simulink model "Simulink_Driver_motor_BLDC"  (R2016a)
settings: Solver=VariableStepAuto  StartTime=0.0  StopTime=0.5  RelTol=1e-3
libraries: powerlib x12, powerlib_meascontrol x1
settings Model: Creator=COMPAQ  LastModifiedBy=COMPAQ

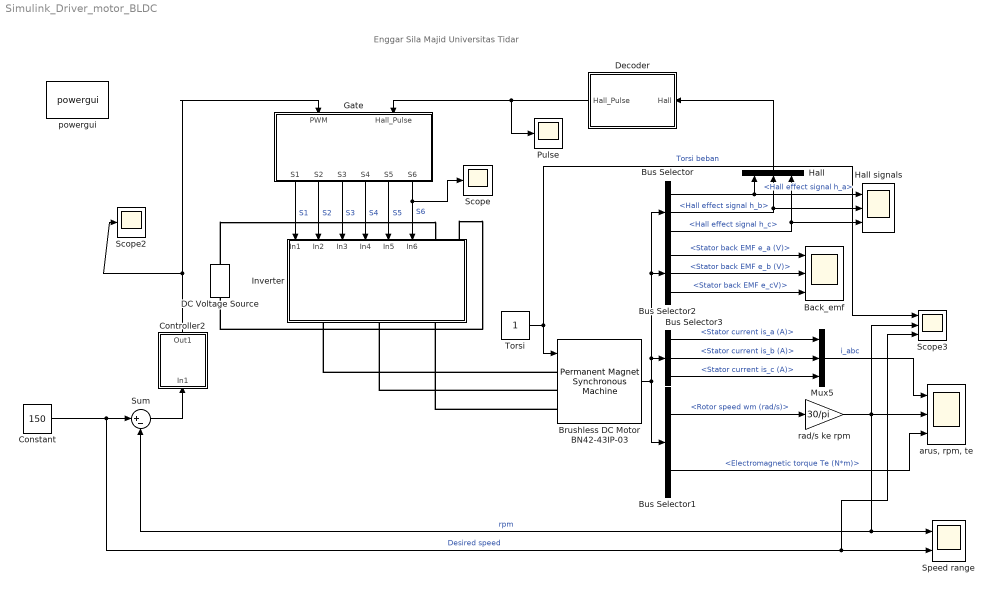
== system Simulink_Driver_motor_BLDC ==
  note: Enggar Sila Majid
      | Universitas Tidar
  Back_emf : Scope  NumInputPorts=3
  Brushless DC Motor BN42-43IP-03 : powerlib/Machines/Permanent Magnet Synchronous Machine  NbPhases=3  FluxDistribution=Trapezoidal  RotorType=Round  MechanicalLoad=Torque Tm  PresetModel=No  ShowDetailedParameters=on  MeasurementBus=off  Resistance=0.16  Inductance=0.00063  dqInductances=[8.5e-3,8.5e-3]  La=0.00126  MachineConstant=Torque Constant (N.m / A_peak)  Flux=0.030319  VoltageCst=25.3998  TorqueCst=0.24255  Flat=120  Mechanical=[0.00036696 0.183593 4]  PolePairs=4  InitialConditions=[0,0, 0,0]  InitialConditions5ph=[0 0 0 0 0 0]  TsPowergui=0  TsBlock=-1  RefAngle=90 degrees behind phase A axis (modified Park)
  Bus Selector : BusSelector  OutputSignals=Hall effect signal h_a,Hall effect signal h_b,Hall effect signal h_c
  Bus Selector1 : BusSelector  OutputSignals=Rotor speed wm (rad/s),Electromagnetic torque Te (N*m)
  Bus Selector2 : BusSelector  OutputSignals=Stator back EMF e_a (V),Stator back EMF e_b (V),Stator back EMF e_cV)
  Bus Selector3 : BusSelector  OutputSignals=Stator current is_a (A),Stator current is_b (A),Stator current is_c (A)
  Constant : Constant  Value=150
  Controller2 : Subsystem
  DC Voltage Source : powerlib/Electrical Sources/DC Voltage Source  Amplitude=48  Measurements=Voltage
  Decoder : Subsystem
  Gate : Subsystem
  Hall : Mux  Inputs=3
  Hall signals : Scope  NumInputPorts=3
  Inverter : Subsystem
  Mux5 : Mux  Inputs=3
  Pulse : Scope
  Scope : Scope
  Scope2 : Scope
  Scope3 : Scope  NumInputPorts=3
  Speed range : Scope  NumInputPorts=2
  Sum : Sum  Inputs=|+-
  Torsi : Constant
  "arus, rpm, te" : Scope  NumInputPorts=3
  powergui : powerlib/powergui  Priority=1  SimulationMode=Discrete  SolverType=Tustin/Backward Euler (TBE)  SampleTime=50e-8  frequency=60  SPID=off  DisableSnubberDevices=off  DisableRonSwitches=off  DisableVfSwitches=off  SwTol=0  DisplayEquations=off  Interpol=off  ExternalGateDelay=off  methode=off  Ts=10  FunctionMessages=off  echomessages=off  HookPort=off  EnableUseOfTLC=off  x0status=blocks  frequencyindice=0  Pbase=100e6  ErrMax=1e-4  Iterations=50  UnitsV=kV  UnitsW=MW  buscounter=0  RestoreLinks=warning  ResistiveCurrentMeasurement=off  Frange=[0:2:500]  Ylog=off  Xlog=on  ShowGrid=off  save=off  variable=ZData  structure=0  ZoomFFT=off  StartTime=0.0  cycles=1  DisplayStyle=1  fundamental=60  FreqAxis=off  MaxFrequency=1000  frequencyindicesteady=1  RmsSteady=1  display=off
  rad/s ke rpm : Gain  Gain=30/pi
  wires:
  Brushless DC Motor BN42-43IP-03/1 -> Bus Selector2/1, Bus Selector/1, Bus Selector3/1, Bus Selector1/1
  Bus Selector1/1 -> rad/s ke rpm/1  "<Rotor speed wm (rad/s)>"
  Bus Selector/2 -> Hall signals/2, Hall/2  "<Hall effect signal h_b>"
  Bus Selector/3 -> Hall signals/3, Hall/3  "<Hall effect signal h_c>"
  Bus Selector1/2 -> "arus, rpm, te"/3  "<Electromagnetic torque Te (N*m)>"
  Bus Selector2/1 -> Back_emf/1  "<Stator back EMF e_a (V)>"
  Bus Selector2/2 -> Back_emf/2  "<Stator back EMF e_b (V)>"
  Bus Selector2/3 -> Back_emf/3  "<Stator back EMF e_cV)>"
  Bus Selector/1 -> Hall signals/1, Hall/1  "<Hall effect signal h_a>"
  Bus Selector3/1 -> Mux5/1  "<Stator current is_a (A)>"
  Bus Selector3/2 -> Mux5/2  "<Stator current is_b (A)>"
  Bus Selector3/3 -> Mux5/3  "<Stator current is_c (A)>"
  Mux5/1 -> "arus, rpm, te"/1  "i_abc"
  Torsi/1 -> Scope3/1, Brushless DC Motor BN42-43IP-03/1  "Torsi beban"
  Hall/1 -> Decoder/1(Hall)
  Gate/1(S1) -> Inverter/1(In1)  "S1"
  Gate/2(S2) -> Inverter/2(In2)  "S2"
  Gate/3(S3) -> Inverter/3(In3)  "S3"
  Gate/4(S4) -> Inverter/4(In4)  "S4"
  Decoder/1(Hall_Pulse) -> Pulse/1, Gate/2(Hall_Pulse)
  Constant/1 -> Scope3/3, Speed range/2, Sum/1  "Desired speed"
  Gate/6(S6) -> Scope/1, Inverter/6(In6)  "S6"
  Gate/5(S5) -> Inverter/5(In5)  "S5"
  rad/s ke rpm/1 -> Scope3/2, Speed range/1, Sum/2, "arus, rpm, te"/2  "rpm"
  Sum/1 -> Controller2/1(In1)
  Controller2/1(Out1) -> Scope2/1, Gate/1(PWM)
  connections:
  Brushless DC Motor BN42-43IP-03/LConn1 -- Inverter/RConn1
  Brushless DC Motor BN42-43IP-03/LConn2 -- Inverter/RConn2
  Brushless DC Motor BN42-43IP-03/LConn3 -- Inverter/RConn3
  DC Voltage Source/RConn1 -- Inverter/LConn1
  Inverter/LConn2 -- DC Voltage Source/LConn1

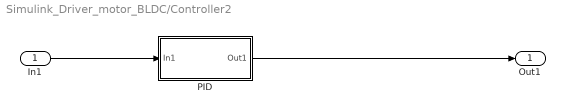
== system Simulink_Driver_motor_BLDC/Controller2 ==
  In1 : Inport
  PID : Subsystem
  Out1 : Outport
  wires:
  PID/1(Out1) -> Out1/1
  In1/1 -> PID/1(In1)

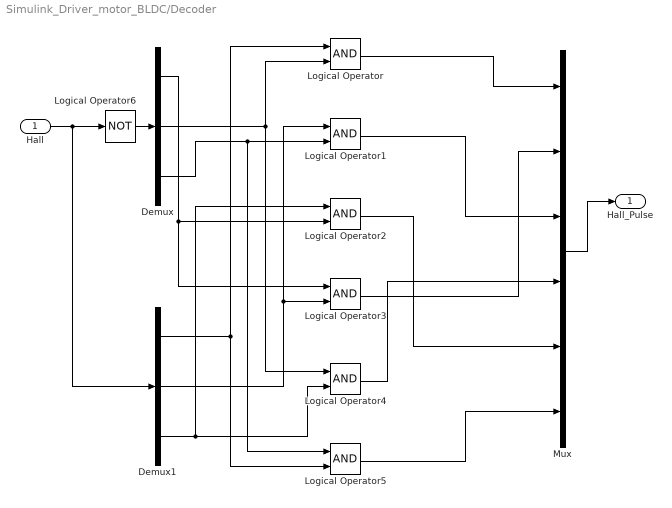
== system Simulink_Driver_motor_BLDC/Decoder ==
  Hall : Inport
  Demux : Demux  Outputs=3
  Demux1 : Demux  Outputs=3
  Logical Operator{,1..5} (6 alike) : Logic  AllPortsSameDT=off  OutDataTypeStr=boolean
  Logical Operator6 : Logic  Operator=NOT  AllPortsSameDT=off  OutDataTypeStr=boolean
  Mux : Mux  Inputs=6
  Hall_Pulse : Outport
  wires:
  Demux1/1 -> Logical Operator/1, Logical Operator5/2
  Demux/2 -> Logical Operator/2, Logical Operator4/1
  Demux1/2 -> Logical Operator3/2, Logical Operator1/1
  Demux/3 -> Logical Operator5/1, Logical Operator1/2
  Demux1/3 -> Logical Operator4/2, Logical Operator2/1
  Demux/1 -> Logical Operator3/1, Logical Operator2/2
  Logical Operator6/1 -> Demux/1
  Hall/1 -> Demux1/1, Logical Operator6/1
  Mux/1 -> Hall_Pulse/1
  Logical Operator/1 -> Mux/1
  Logical Operator1/1 -> Mux/3
  Logical Operator2/1 -> Mux/5
  Logical Operator3/1 -> Mux/2
  Logical Operator4/1 -> Mux/4
  Logical Operator5/1 -> Mux/6

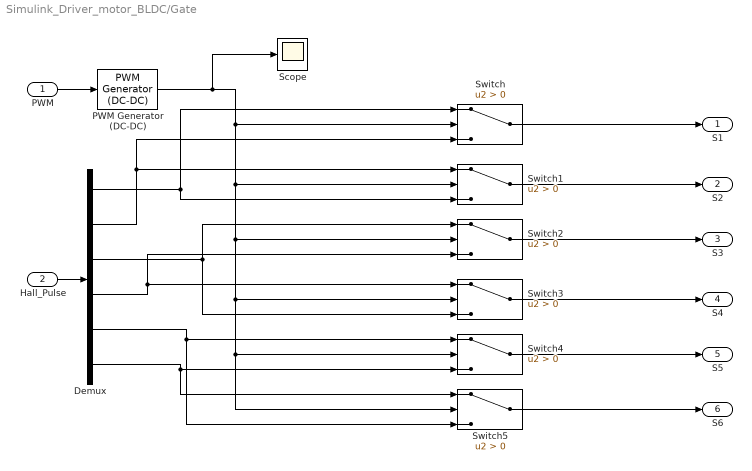
== system Simulink_Driver_motor_BLDC/Gate ==
  PWM : Inport
  Hall_Pulse : Inport  Port=2
  Demux : Demux  Outputs=6
  PWM Generator (DC-DC) : powerlib_meascontrol/Pulse & Signal Generators/PWM Generator (DC-DC)  Fsw=50  Ts=0
  Scope : Scope
  Switch{,1..5} (6 alike) : Switch  Criteria=u2 > Threshold
  S1 : Outport
  S2 : Outport  Port=2
  S3 : Outport  Port=3
  S4 : Outport  Port=4
  S5 : Outport  Port=5
  S6 : Outport  Port=6
  wires:
  Hall_Pulse/1 -> Demux/1
  Demux/1 -> Switch1/3, Switch/1
  Demux/2 -> Switch1/1, Switch/3
  Demux/3 -> Switch3/3, Switch2/1
  Demux/4 -> Switch3/1, Switch2/3
  Demux/5 -> Switch5/3, Switch4/1
  Demux/6 -> Switch5/1, Switch4/3
  PWM/1 -> PWM Generator (DC-DC)/1
  Switch/1 -> S1/1
  Switch1/1 -> S2/1
  Switch2/1 -> S3/1
  Switch3/1 -> S4/1
  Switch4/1 -> S5/1
  Switch5/1 -> S6/1
  PWM Generator (DC-DC)/1 -> Scope/1, Switch/2, Switch1/2, Switch2/2, Switch3/2, Switch5/2, Switch4/2

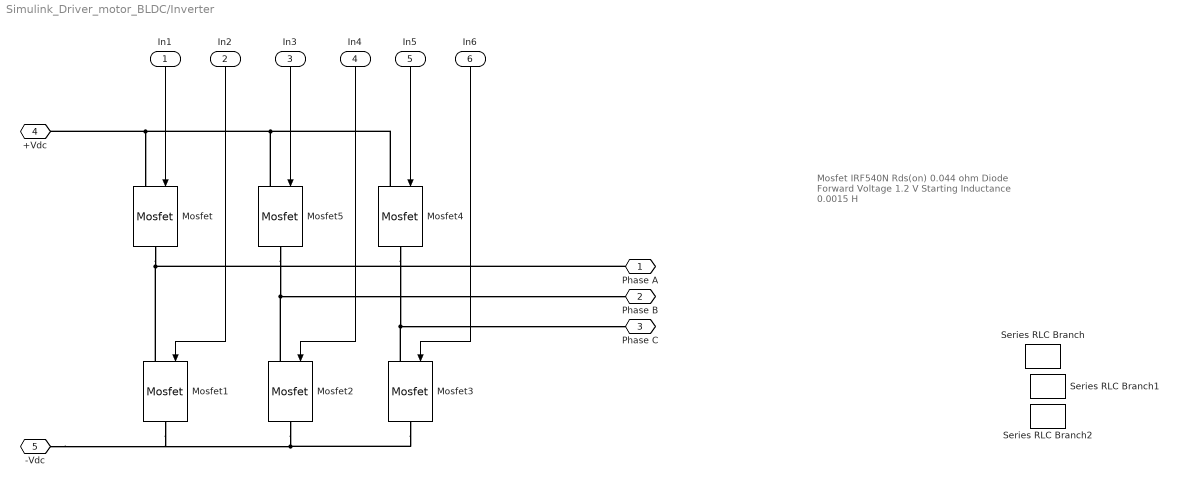
== system Simulink_Driver_motor_BLDC/Inverter ==
  note: Mosfet IRF540N
      |
      | Rds(on)
      | 0.044 ohm
      |
      | Diode Forward Voltage
      | 1.2 V
      |
      | Starting Inductance
      | 0.0015 H
  In1 : Inport  OutMax=[1]
  In2 : Inport  Port=2  OutMax=[1]
  In3 : Inport  Port=3  OutMax=[1]
  In4 : Inport  Port=4  OutMax=[1]
  In5 : Inport  Port=5  OutMax=[1]
  In6 : Inport  Port=6  OutMax=[1]
  Mosfet{,1..5} (6 alike) : powerlib/Power Electronics/Mosfet  Ron=0.044  Lon=0.0015  Rd=0.044  Vfd=1.2  IC=0  Rs=0.044  Cs=12  Measurements=off
  Series RLC Branch : powerlib/Elements/Series RLC Branch  LConnTagsString=__new0  RConnTagsString=__new0  BranchType=R  Resistance=0.0015  Inductance=1e-3  SetiL0=off  InitialCurrent=0  Capacitance=1e-6  Setx0=off  InitialVoltage=0  Measurements=Branch current
  Series RLC Branch1 : powerlib/Elements/Series RLC Branch  LConnTagsString=__new0  RConnTagsString=__new0  BranchType=R  Resistance=0.0015  Inductance=1e-3  SetiL0=off  InitialCurrent=0  Capacitance=1e-6  Setx0=off  InitialVoltage=0  Measurements=Branch current
  Series RLC Branch2 : powerlib/Elements/Series RLC Branch  LConnTagsString=__new0  RConnTagsString=__new0  BranchType=R  Resistance=0.0015  Inductance=1e-3  SetiL0=off  InitialCurrent=0  Capacitance=1e-6  Setx0=off  InitialVoltage=0  Measurements=Branch current
  Phase A : PMIOPort  Port=1  Side=Right
  Phase B : PMIOPort  Port=2  Side=Right
  Phase C : PMIOPort  Port=3  Side=Right
  +Vdc : PMIOPort  Port=4  Side=Left
  -Vdc : PMIOPort  Port=5  Side=Left
  wires:
  In4/1 -> Mosfet2/1
  In6/1 -> Mosfet3/1
  In3/1 -> Mosfet5/1
  In2/1 -> Mosfet1/1
  In1/1 -> Mosfet/1
  In5/1 -> Mosfet4/1
  connections:
  Mosfet4/LConn1 -- Mosfet5/LConn1 -- +Vdc/RConn1 -- Mosfet/LConn1
  Mosfet2/RConn1 -- Mosfet3/RConn1 -- -Vdc/RConn1 -- Mosfet1/RConn1
  Mosfet/RConn1 -- Phase A/RConn1 -- Mosfet1/LConn1
  Mosfet5/RConn1 -- Phase B/RConn1 -- Mosfet2/LConn1
  Mosfet4/RConn1 -- Phase C/RConn1 -- Mosfet3/LConn1

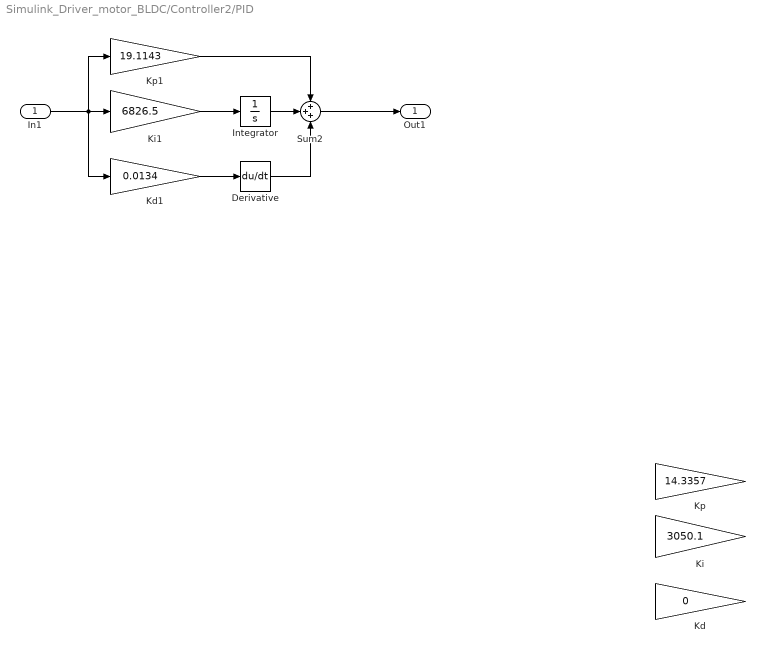
== system Simulink_Driver_motor_BLDC/Controller2/PID ==
  In1 : Inport
  Derivative : Derivative
  Integrator : Integrator
  Kd : Gain  Gain=0
  Kd1 : Gain  Gain=0.0134
  Ki : Gain  Gain=3050.1
  Ki1 : Gain  Gain=6826.5
  Kp : Gain  Gain=14.3357
  Kp1 : Gain  Gain=19.1143
  Sum2 : Sum  Inputs=+++
  Out1 : Outport
  wires:
  Sum2/1 -> Out1/1
  Kp1/1 -> Sum2/1
  In1/1 -> Kd1/1, Ki1/1, Kp1/1
  Kd1/1 -> Derivative/1
  Ki1/1 -> Integrator/1
  Integrator/1 -> Sum2/2
  Derivative/1 -> Sum2/3
